simulink model "bit32cpu"  (R2020a)
settings: Solver=VariableStepAuto  StartTime=0.0  StopTime=10.0  RelTol=1e-3
libraries: simulink_extras x392
(part 7 of 63)

== system bit32cpu/ALU/Subsystem7/Subsystem2/Subsystem1 ==
  In1 : Inport
  In2 : Inport  Port=2
  In3 : Inport  Port=3
  In4 : Inport  Port=4
  In5 : Inport  Port=5
  In7 : Inport  Port=6
  In6 : Inport  Port=7
  Demux{,1..3} (4 alike) : Demux  Outputs=8
  Mux : Mux  Inputs=8
  Subsystem : Subsystem
  Subsystem1 : Subsystem
  Subsystem2 : Subsystem
  Subsystem3 : Subsystem
  Subsystem4 : Subsystem
  Subsystem5 : Subsystem
  Subsystem6 : Subsystem
  Subsystem7 : Subsystem
  Out1 : Outport
  wires:
  Demux3/7 -> Subsystem6/6(In6)
  In6/1 -> Subsystem4/7(In7), Subsystem7/7(In7), Subsystem5/7(In7), Subsystem6/7(In7), Subsystem1/7(In7), Subsystem3/7(In7), Subsystem2/7(In7), Subsystem/7(In7)
  Subsystem3/1(Out1) -> Mux/4
  Demux/1 -> Subsystem/3(In3)
  Demux2/8 -> Subsystem7/5(In5)
  Subsystem1/1(Out1) -> Mux/2
  Subsystem2/1(Out1) -> Mux/3
  Subsystem4/1(Out1) -> Mux/5
  Demux1/2 -> Subsystem1/4(In4)
  Demux/6 -> Subsystem5/3(In3)
  In4/1 -> Demux1/1
  Demux2/7 -> Subsystem6/5(In5)
  In3/1 -> Demux/1
  Demux1/4 -> Subsystem3/4(In4)
  In2/1 -> Subsystem4/2(In2), Subsystem5/2(In2), Subsystem6/2(In2), Subsystem7/2(In2), Subsystem2/2(In2), Subsystem3/2(In2), Subsystem/2(In2), Subsystem1/2(In2)
  Demux3/3 -> Subsystem2/6(In6)
  Subsystem/1(Out1) -> Mux/1
  Subsystem5/1(Out1) -> Mux/6
  In7/1 -> Demux3/1
  Mux/1 -> Out1/1
  Demux/3 -> Subsystem2/3(In3)
  Demux1/8 -> Subsystem7/4(In4)
  Demux3/6 -> Subsystem5/6(In6)
  Demux3/1 -> Subsystem/6(In6)
  Demux3/2 -> Subsystem1/6(In6)
  Subsystem6/1(Out1) -> Mux/7
  Demux1/3 -> Subsystem2/4(In4)
  Demux2/4 -> Subsystem3/5(In5)
  Demux1/5 -> Subsystem4/4(In4)
  In1/1 -> Subsystem6/1(In1), Subsystem7/1(In1), Subsystem4/1(In1), Subsystem5/1(In1), Subsystem2/1(In1), Subsystem3/1(In1), Subsystem/1(In1), Subsystem1/1(In1)
  Demux1/1 -> Subsystem/4(In4)
  Demux3/4 -> Subsystem3/6(In6)
  Demux2/2 -> Subsystem1/5(In5)
  Demux2/6 -> Subsystem5/5(In5)
  Demux/2 -> Subsystem1/3(In3)
  Demux/7 -> Subsystem6/3(In3)
  Demux3/8 -> Subsystem7/6(In6)
  Demux1/6 -> Subsystem5/4(In4)
  Demux/5 -> Subsystem4/3(In3)
  Demux2/5 -> Subsystem4/5(In5)
  Demux/8 -> Subsystem7/3(In3)
  Demux2/3 -> Subsystem2/5(In5)
  Demux3/5 -> Subsystem4/6(In6)
  In5/1 -> Demux2/1
  Demux1/7 -> Subsystem6/4(In4)
  Subsystem7/1(Out1) -> Mux/8
  Demux/4 -> Subsystem3/3(In3)
  Demux2/1 -> Subsystem/5(In5)

== system bit32cpu/ALU/Subsystem7/Subsystem2/Subsystem2 ==
  In1 : Inport
  In2 : Inport  Port=2
  In3 : Inport  Port=3
  In4 : Inport  Port=4
  In5 : Inport  Port=5
  In7 : Inport  Port=6
  In6 : Inport  Port=7
  Demux{,1..3} (4 alike) : Demux  Outputs=8
  Mux : Mux  Inputs=8
  Subsystem : Subsystem
  Subsystem1 : Subsystem
  Subsystem2 : Subsystem
  Subsystem3 : Subsystem
  Subsystem4 : Subsystem
  Subsystem5 : Subsystem
  Subsystem6 : Subsystem
  Subsystem7 : Subsystem
  Out1 : Outport
  wires:
  Demux3/7 -> Subsystem6/6(In6)
  In6/1 -> Subsystem4/7(In7), Subsystem7/7(In7), Subsystem5/7(In7), Subsystem6/7(In7), Subsystem1/7(In7), Subsystem3/7(In7), Subsystem2/7(In7), Subsystem/7(In7)
  Subsystem3/1(Out1) -> Mux/4
  Demux/1 -> Subsystem/3(In3)
  Demux2/8 -> Subsystem7/5(In5)
  Subsystem1/1(Out1) -> Mux/2
  Subsystem2/1(Out1) -> Mux/3
  Subsystem4/1(Out1) -> Mux/5
  Demux1/2 -> Subsystem1/4(In4)
  Demux/6 -> Subsystem5/3(In3)
  In4/1 -> Demux1/1
  Demux2/7 -> Subsystem6/5(In5)
  In3/1 -> Demux/1
  Demux1/4 -> Subsystem3/4(In4)
  In2/1 -> Subsystem4/2(In2), Subsystem5/2(In2), Subsystem6/2(In2), Subsystem7/2(In2), Subsystem2/2(In2), Subsystem3/2(In2), Subsystem/2(In2), Subsystem1/2(In2)
  Demux3/3 -> Subsystem2/6(In6)
  Subsystem/1(Out1) -> Mux/1
  Subsystem5/1(Out1) -> Mux/6
  In7/1 -> Demux3/1
  Mux/1 -> Out1/1
  Demux/3 -> Subsystem2/3(In3)
  Demux1/8 -> Subsystem7/4(In4)
  Demux3/6 -> Subsystem5/6(In6)
  Demux3/1 -> Subsystem/6(In6)
  Demux3/2 -> Subsystem1/6(In6)
  Subsystem6/1(Out1) -> Mux/7
  Demux1/3 -> Subsystem2/4(In4)
  Demux2/4 -> Subsystem3/5(In5)
  Demux1/5 -> Subsystem4/4(In4)
  In1/1 -> Subsystem6/1(In1), Subsystem7/1(In1), Subsystem4/1(In1), Subsystem5/1(In1), Subsystem2/1(In1), Subsystem3/1(In1), Subsystem/1(In1), Subsystem1/1(In1)
  Demux1/1 -> Subsystem/4(In4)
  Demux3/4 -> Subsystem3/6(In6)
  Demux2/2 -> Subsystem1/5(In5)
  Demux2/6 -> Subsystem5/5(In5)
  Demux/2 -> Subsystem1/3(In3)
  Demux/7 -> Subsystem6/3(In3)
  Demux3/8 -> Subsystem7/6(In6)
  Demux1/6 -> Subsystem5/4(In4)
  Demux/5 -> Subsystem4/3(In3)
  Demux2/5 -> Subsystem4/5(In5)
  Demux/8 -> Subsystem7/3(In3)
  Demux2/3 -> Subsystem2/5(In5)
  Demux3/5 -> Subsystem4/6(In6)
  In5/1 -> Demux2/1
  Demux1/7 -> Subsystem6/4(In4)
  Subsystem7/1(Out1) -> Mux/8
  Demux/4 -> Subsystem3/3(In3)
  Demux2/1 -> Subsystem/5(In5)

== system bit32cpu/ALU/Subsystem7/Subsystem2/Subsystem3 ==
  In1 : Inport
  In2 : Inport  Port=2
  In3 : Inport  Port=3
  In4 : Inport  Port=4
  In5 : Inport  Port=5
  In7 : Inport  Port=6
  In6 : Inport  Port=7
  Demux{,1..3} (4 alike) : Demux  Outputs=8
  Mux : Mux  Inputs=8
  Subsystem : Subsystem
  Subsystem1 : Subsystem
  Subsystem2 : Subsystem
  Subsystem3 : Subsystem
  Subsystem4 : Subsystem
  Subsystem5 : Subsystem
  Subsystem6 : Subsystem
  Subsystem7 : Subsystem
  Out1 : Outport
  wires:
  Demux3/7 -> Subsystem6/6(In6)
  In6/1 -> Subsystem4/7(In7), Subsystem7/7(In7), Subsystem5/7(In7), Subsystem6/7(In7), Subsystem1/7(In7), Subsystem3/7(In7), Subsystem2/7(In7), Subsystem/7(In7)
  Subsystem3/1(Out1) -> Mux/4
  Demux/1 -> Subsystem/3(In3)
  Demux2/8 -> Subsystem7/5(In5)
  Subsystem1/1(Out1) -> Mux/2
  Subsystem2/1(Out1) -> Mux/3
  Subsystem4/1(Out1) -> Mux/5
  Demux1/2 -> Subsystem1/4(In4)
  Demux/6 -> Subsystem5/3(In3)
  In4/1 -> Demux1/1
  Demux2/7 -> Subsystem6/5(In5)
  In3/1 -> Demux/1
  Demux1/4 -> Subsystem3/4(In4)
  In2/1 -> Subsystem4/2(In2), Subsystem5/2(In2), Subsystem6/2(In2), Subsystem7/2(In2), Subsystem2/2(In2), Subsystem3/2(In2), Subsystem/2(In2), Subsystem1/2(In2)
  Demux3/3 -> Subsystem2/6(In6)
  Subsystem/1(Out1) -> Mux/1
  Subsystem5/1(Out1) -> Mux/6
  In7/1 -> Demux3/1
  Mux/1 -> Out1/1
  Demux/3 -> Subsystem2/3(In3)
  Demux1/8 -> Subsystem7/4(In4)
  Demux3/6 -> Subsystem5/6(In6)
  Demux3/1 -> Subsystem/6(In6)
  Demux3/2 -> Subsystem1/6(In6)
  Subsystem6/1(Out1) -> Mux/7
  Demux1/3 -> Subsystem2/4(In4)
  Demux2/4 -> Subsystem3/5(In5)
  Demux1/5 -> Subsystem4/4(In4)
  In1/1 -> Subsystem6/1(In1), Subsystem7/1(In1), Subsystem4/1(In1), Subsystem5/1(In1), Subsystem2/1(In1), Subsystem3/1(In1), Subsystem/1(In1), Subsystem1/1(In1)
  Demux1/1 -> Subsystem/4(In4)
  Demux3/4 -> Subsystem3/6(In6)
  Demux2/2 -> Subsystem1/5(In5)
  Demux2/6 -> Subsystem5/5(In5)
  Demux/2 -> Subsystem1/3(In3)
  Demux/7 -> Subsystem6/3(In3)
  Demux3/8 -> Subsystem7/6(In6)
  Demux1/6 -> Subsystem5/4(In4)
  Demux/5 -> Subsystem4/3(In3)
  Demux2/5 -> Subsystem4/5(In5)
  Demux/8 -> Subsystem7/3(In3)
  Demux2/3 -> Subsystem2/5(In5)
  Demux3/5 -> Subsystem4/6(In6)
  In5/1 -> Demux2/1
  Demux1/7 -> Subsystem6/4(In4)
  Subsystem7/1(Out1) -> Mux/8
  Demux/4 -> Subsystem3/3(In3)
  Demux2/1 -> Subsystem/5(In5)

== system bit32cpu/ALU/Subsystem7/Subsystem2/Subsystem4 ==
  In1 : Inport
  In2 : Inport  Port=2
  In3 : Inport  Port=3
  In4 : Inport  Port=4
  In5 : Inport  Port=5
  In7 : Inport  Port=6
  In6 : Inport  Port=7
  Demux{,1..3} (4 alike) : Demux  Outputs=8
  Mux : Mux  Inputs=8
  Subsystem : Subsystem
  Subsystem1 : Subsystem
  Subsystem2 : Subsystem
  Subsystem3 : Subsystem
  Subsystem4 : Subsystem
  Subsystem5 : Subsystem
  Subsystem6 : Subsystem
  Subsystem7 : Subsystem
  Out1 : Outport
  wires:
  Demux3/7 -> Subsystem6/6(In6)
  In6/1 -> Subsystem4/7(In7), Subsystem7/7(In7), Subsystem5/7(In7), Subsystem6/7(In7), Subsystem1/7(In7), Subsystem3/7(In7), Subsystem2/7(In7), Subsystem/7(In7)
  Subsystem3/1(Out1) -> Mux/4
  Demux/1 -> Subsystem/3(In3)
  Demux2/8 -> Subsystem7/5(In5)
  Subsystem1/1(Out1) -> Mux/2
  Subsystem2/1(Out1) -> Mux/3
  Subsystem4/1(Out1) -> Mux/5
  Demux1/2 -> Subsystem1/4(In4)
  Demux/6 -> Subsystem5/3(In3)
  In4/1 -> Demux1/1
  Demux2/7 -> Subsystem6/5(In5)
  In3/1 -> Demux/1
  Demux1/4 -> Subsystem3/4(In4)
  In2/1 -> Subsystem4/2(In2), Subsystem5/2(In2), Subsystem6/2(In2), Subsystem7/2(In2), Subsystem2/2(In2), Subsystem3/2(In2), Subsystem/2(In2), Subsystem1/2(In2)
  Demux3/3 -> Subsystem2/6(In6)
  Subsystem/1(Out1) -> Mux/1
  Subsystem5/1(Out1) -> Mux/6
  In7/1 -> Demux3/1
  Mux/1 -> Out1/1
  Demux/3 -> Subsystem2/3(In3)
  Demux1/8 -> Subsystem7/4(In4)
  Demux3/6 -> Subsystem5/6(In6)
  Demux3/1 -> Subsystem/6(In6)
  Demux3/2 -> Subsystem1/6(In6)
  Subsystem6/1(Out1) -> Mux/7
  Demux1/3 -> Subsystem2/4(In4)
  Demux2/4 -> Subsystem3/5(In5)
  Demux1/5 -> Subsystem4/4(In4)
  In1/1 -> Subsystem6/1(In1), Subsystem7/1(In1), Subsystem4/1(In1), Subsystem5/1(In1), Subsystem2/1(In1), Subsystem3/1(In1), Subsystem/1(In1), Subsystem1/1(In1)
  Demux1/1 -> Subsystem/4(In4)
  Demux3/4 -> Subsystem3/6(In6)
  Demux2/2 -> Subsystem1/5(In5)
  Demux2/6 -> Subsystem5/5(In5)
  Demux/2 -> Subsystem1/3(In3)
  Demux/7 -> Subsystem6/3(In3)
  Demux3/8 -> Subsystem7/6(In6)
  Demux1/6 -> Subsystem5/4(In4)
  Demux/5 -> Subsystem4/3(In3)
  Demux2/5 -> Subsystem4/5(In5)
  Demux/8 -> Subsystem7/3(In3)
  Demux2/3 -> Subsystem2/5(In5)
  Demux3/5 -> Subsystem4/6(In6)
  In5/1 -> Demux2/1
  Demux1/7 -> Subsystem6/4(In4)
  Subsystem7/1(Out1) -> Mux/8
  Demux/4 -> Subsystem3/3(In3)
  Demux2/1 -> Subsystem/5(In5)

== system bit32cpu/ALU/Subsystem7/Subsystem2/Subsystem5 ==
  In1 : Inport
  In2 : Inport  Port=2
  In3 : Inport  Port=3
  In4 : Inport  Port=4
  In5 : Inport  Port=5
  In7 : Inport  Port=6
  In6 : Inport  Port=7
  Demux{,1..3} (4 alike) : Demux  Outputs=8
  Mux : Mux  Inputs=8
  Subsystem : Subsystem
  Subsystem1 : Subsystem
  Subsystem2 : Subsystem
  Subsystem3 : Subsystem
  Subsystem4 : Subsystem
  Subsystem5 : Subsystem
  Subsystem6 : Subsystem
  Subsystem7 : Subsystem
  Out1 : Outport
  wires:
  Demux3/7 -> Subsystem6/6(In6)
  In6/1 -> Subsystem4/7(In7), Subsystem7/7(In7), Subsystem5/7(In7), Subsystem6/7(In7), Subsystem1/7(In7), Subsystem3/7(In7), Subsystem2/7(In7), Subsystem/7(In7)
  Subsystem3/1(Out1) -> Mux/4
  Demux/1 -> Subsystem/3(In3)
  Demux2/8 -> Subsystem7/5(In5)
  Subsystem1/1(Out1) -> Mux/2
  Subsystem2/1(Out1) -> Mux/3
  Subsystem4/1(Out1) -> Mux/5
  Demux1/2 -> Subsystem1/4(In4)
  Demux/6 -> Subsystem5/3(In3)
  In4/1 -> Demux1/1
  Demux2/7 -> Subsystem6/5(In5)
  In3/1 -> Demux/1
  Demux1/4 -> Subsystem3/4(In4)
  In2/1 -> Subsystem4/2(In2), Subsystem5/2(In2), Subsystem6/2(In2), Subsystem7/2(In2), Subsystem2/2(In2), Subsystem3/2(In2), Subsystem/2(In2), Subsystem1/2(In2)
  Demux3/3 -> Subsystem2/6(In6)
  Subsystem/1(Out1) -> Mux/1
  Subsystem5/1(Out1) -> Mux/6
  In7/1 -> Demux3/1
  Mux/1 -> Out1/1
  Demux/3 -> Subsystem2/3(In3)
  Demux1/8 -> Subsystem7/4(In4)
  Demux3/6 -> Subsystem5/6(In6)
  Demux3/1 -> Subsystem/6(In6)
  Demux3/2 -> Subsystem1/6(In6)
  Subsystem6/1(Out1) -> Mux/7
  Demux1/3 -> Subsystem2/4(In4)
  Demux2/4 -> Subsystem3/5(In5)
  Demux1/5 -> Subsystem4/4(In4)
  In1/1 -> Subsystem6/1(In1), Subsystem7/1(In1), Subsystem4/1(In1), Subsystem5/1(In1), Subsystem2/1(In1), Subsystem3/1(In1), Subsystem/1(In1), Subsystem1/1(In1)
  Demux1/1 -> Subsystem/4(In4)
  Demux3/4 -> Subsystem3/6(In6)
  Demux2/2 -> Subsystem1/5(In5)
  Demux2/6 -> Subsystem5/5(In5)
  Demux/2 -> Subsystem1/3(In3)
  Demux/7 -> Subsystem6/3(In3)
  Demux3/8 -> Subsystem7/6(In6)
  Demux1/6 -> Subsystem5/4(In4)
  Demux/5 -> Subsystem4/3(In3)
  Demux2/5 -> Subsystem4/5(In5)
  Demux/8 -> Subsystem7/3(In3)
  Demux2/3 -> Subsystem2/5(In5)
  Demux3/5 -> Subsystem4/6(In6)
  In5/1 -> Demux2/1
  Demux1/7 -> Subsystem6/4(In4)
  Subsystem7/1(Out1) -> Mux/8
  Demux/4 -> Subsystem3/3(In3)
  Demux2/1 -> Subsystem/5(In5)

== system bit32cpu/ALU/Subsystem7/Subsystem3/Subsystem1 ==
  In1 : Inport
  In2 : Inport  Port=2
  In3 : Inport  Port=3
  In4 : Inport  Port=4
  In5 : Inport  Port=5
  In7 : Inport  Port=6
  In6 : Inport  Port=7
  Demux{,1..3} (4 alike) : Demux  Outputs=8
  Mux : Mux  Inputs=8
  Subsystem : Subsystem
  Subsystem1 : Subsystem
  Subsystem2 : Subsystem
  Subsystem3 : Subsystem
  Subsystem4 : Subsystem
  Subsystem5 : Subsystem
  Subsystem6 : Subsystem
  Subsystem7 : Subsystem
  Out1 : Outport
  wires:
  Demux3/7 -> Subsystem6/6(In6)
  In6/1 -> Subsystem4/7(In7), Subsystem7/7(In7), Subsystem5/7(In7), Subsystem6/7(In7), Subsystem1/7(In7), Subsystem3/7(In7), Subsystem2/7(In7), Subsystem/7(In7)
  Subsystem3/1(Out1) -> Mux/4
  Demux/1 -> Subsystem/3(In3)
  Demux2/8 -> Subsystem7/5(In5)
  Subsystem1/1(Out1) -> Mux/2
  Subsystem2/1(Out1) -> Mux/3
  Subsystem4/1(Out1) -> Mux/5
  Demux1/2 -> Subsystem1/4(In4)
  Demux/6 -> Subsystem5/3(In3)
  In4/1 -> Demux1/1
  Demux2/7 -> Subsystem6/5(In5)
  In3/1 -> Demux/1
  Demux1/4 -> Subsystem3/4(In4)
  In2/1 -> Subsystem4/2(In2), Subsystem5/2(In2), Subsystem6/2(In2), Subsystem7/2(In2), Subsystem2/2(In2), Subsystem3/2(In2), Subsystem/2(In2), Subsystem1/2(In2)
  Demux3/3 -> Subsystem2/6(In6)
  Subsystem/1(Out1) -> Mux/1
  Subsystem5/1(Out1) -> Mux/6
  In7/1 -> Demux3/1
  Mux/1 -> Out1/1
  Demux/3 -> Subsystem2/3(In3)
  Demux1/8 -> Subsystem7/4(In4)
  Demux3/6 -> Subsystem5/6(In6)
  Demux3/1 -> Subsystem/6(In6)
  Demux3/2 -> Subsystem1/6(In6)
  Subsystem6/1(Out1) -> Mux/7
  Demux1/3 -> Subsystem2/4(In4)
  Demux2/4 -> Subsystem3/5(In5)
  Demux1/5 -> Subsystem4/4(In4)
  In1/1 -> Subsystem6/1(In1), Subsystem7/1(In1), Subsystem4/1(In1), Subsystem5/1(In1), Subsystem2/1(In1), Subsystem3/1(In1), Subsystem/1(In1), Subsystem1/1(In1)
  Demux1/1 -> Subsystem/4(In4)
  Demux3/4 -> Subsystem3/6(In6)
  Demux2/2 -> Subsystem1/5(In5)
  Demux2/6 -> Subsystem5/5(In5)
  Demux/2 -> Subsystem1/3(In3)
  Demux/7 -> Subsystem6/3(In3)
  Demux3/8 -> Subsystem7/6(In6)
  Demux1/6 -> Subsystem5/4(In4)
  Demux/5 -> Subsystem4/3(In3)
  Demux2/5 -> Subsystem4/5(In5)
  Demux/8 -> Subsystem7/3(In3)
  Demux2/3 -> Subsystem2/5(In5)
  Demux3/5 -> Subsystem4/6(In6)
  In5/1 -> Demux2/1
  Demux1/7 -> Subsystem6/4(In4)
  Subsystem7/1(Out1) -> Mux/8
  Demux/4 -> Subsystem3/3(In3)
  Demux2/1 -> Subsystem/5(In5)

== system bit32cpu/ALU/Subsystem7/Subsystem3/Subsystem2 ==
  In1 : Inport
  In2 : Inport  Port=2
  In3 : Inport  Port=3
  In4 : Inport  Port=4
  In5 : Inport  Port=5
  In7 : Inport  Port=6
  In6 : Inport  Port=7
  Demux{,1..3} (4 alike) : Demux  Outputs=8
  Mux : Mux  Inputs=8
  Subsystem : Subsystem
  Subsystem1 : Subsystem
  Subsystem2 : Subsystem
  Subsystem3 : Subsystem
  Subsystem4 : Subsystem
  Subsystem5 : Subsystem
  Subsystem6 : Subsystem
  Subsystem7 : Subsystem
  Out1 : Outport
  wires:
  Demux3/7 -> Subsystem6/6(In6)
  In6/1 -> Subsystem4/7(In7), Subsystem7/7(In7), Subsystem5/7(In7), Subsystem6/7(In7), Subsystem1/7(In7), Subsystem3/7(In7), Subsystem2/7(In7), Subsystem/7(In7)
  Subsystem3/1(Out1) -> Mux/4
  Demux/1 -> Subsystem/3(In3)
  Demux2/8 -> Subsystem7/5(In5)
  Subsystem1/1(Out1) -> Mux/2
  Subsystem2/1(Out1) -> Mux/3
  Subsystem4/1(Out1) -> Mux/5
  Demux1/2 -> Subsystem1/4(In4)
  Demux/6 -> Subsystem5/3(In3)
  In4/1 -> Demux1/1
  Demux2/7 -> Subsystem6/5(In5)
  In3/1 -> Demux/1
  Demux1/4 -> Subsystem3/4(In4)
  In2/1 -> Subsystem4/2(In2), Subsystem5/2(In2), Subsystem6/2(In2), Subsystem7/2(In2), Subsystem2/2(In2), Subsystem3/2(In2), Subsystem/2(In2), Subsystem1/2(In2)
  Demux3/3 -> Subsystem2/6(In6)
  Subsystem/1(Out1) -> Mux/1
  Subsystem5/1(Out1) -> Mux/6
  In7/1 -> Demux3/1
  Mux/1 -> Out1/1
  Demux/3 -> Subsystem2/3(In3)
  Demux1/8 -> Subsystem7/4(In4)
  Demux3/6 -> Subsystem5/6(In6)
  Demux3/1 -> Subsystem/6(In6)
  Demux3/2 -> Subsystem1/6(In6)
  Subsystem6/1(Out1) -> Mux/7
  Demux1/3 -> Subsystem2/4(In4)
  Demux2/4 -> Subsystem3/5(In5)
  Demux1/5 -> Subsystem4/4(In4)
  In1/1 -> Subsystem6/1(In1), Subsystem7/1(In1), Subsystem4/1(In1), Subsystem5/1(In1), Subsystem2/1(In1), Subsystem3/1(In1), Subsystem/1(In1), Subsystem1/1(In1)
  Demux1/1 -> Subsystem/4(In4)
  Demux3/4 -> Subsystem3/6(In6)
  Demux2/2 -> Subsystem1/5(In5)
  Demux2/6 -> Subsystem5/5(In5)
  Demux/2 -> Subsystem1/3(In3)
  Demux/7 -> Subsystem6/3(In3)
  Demux3/8 -> Subsystem7/6(In6)
  Demux1/6 -> Subsystem5/4(In4)
  Demux/5 -> Subsystem4/3(In3)
  Demux2/5 -> Subsystem4/5(In5)
  Demux/8 -> Subsystem7/3(In3)
  Demux2/3 -> Subsystem2/5(In5)
  Demux3/5 -> Subsystem4/6(In6)
  In5/1 -> Demux2/1
  Demux1/7 -> Subsystem6/4(In4)
  Subsystem7/1(Out1) -> Mux/8
  Demux/4 -> Subsystem3/3(In3)
  Demux2/1 -> Subsystem/5(In5)

== system bit32cpu/ALU/Subsystem7/Subsystem3/Subsystem3 ==
  In1 : Inport
  In2 : Inport  Port=2
  In3 : Inport  Port=3
  In4 : Inport  Port=4
  In5 : Inport  Port=5
  In7 : Inport  Port=6
  In6 : Inport  Port=7
  Demux{,1..3} (4 alike) : Demux  Outputs=8
  Mux : Mux  Inputs=8
  Subsystem : Subsystem
  Subsystem1 : Subsystem
  Subsystem2 : Subsystem
  Subsystem3 : Subsystem
  Subsystem4 : Subsystem
  Subsystem5 : Subsystem
  Subsystem6 : Subsystem
  Subsystem7 : Subsystem
  Out1 : Outport
  wires:
  Demux3/7 -> Subsystem6/6(In6)
  In6/1 -> Subsystem4/7(In7), Subsystem7/7(In7), Subsystem5/7(In7), Subsystem6/7(In7), Subsystem1/7(In7), Subsystem3/7(In7), Subsystem2/7(In7), Subsystem/7(In7)
  Subsystem3/1(Out1) -> Mux/4
  Demux/1 -> Subsystem/3(In3)
  Demux2/8 -> Subsystem7/5(In5)
  Subsystem1/1(Out1) -> Mux/2
  Subsystem2/1(Out1) -> Mux/3
  Subsystem4/1(Out1) -> Mux/5
  Demux1/2 -> Subsystem1/4(In4)
  Demux/6 -> Subsystem5/3(In3)
  In4/1 -> Demux1/1
  Demux2/7 -> Subsystem6/5(In5)
  In3/1 -> Demux/1
  Demux1/4 -> Subsystem3/4(In4)
  In2/1 -> Subsystem4/2(In2), Subsystem5/2(In2), Subsystem6/2(In2), Subsystem7/2(In2), Subsystem2/2(In2), Subsystem3/2(In2), Subsystem/2(In2), Subsystem1/2(In2)
  Demux3/3 -> Subsystem2/6(In6)
  Subsystem/1(Out1) -> Mux/1
  Subsystem5/1(Out1) -> Mux/6
  In7/1 -> Demux3/1
  Mux/1 -> Out1/1
  Demux/3 -> Subsystem2/3(In3)
  Demux1/8 -> Subsystem7/4(In4)
  Demux3/6 -> Subsystem5/6(In6)
  Demux3/1 -> Subsystem/6(In6)
  Demux3/2 -> Subsystem1/6(In6)
  Subsystem6/1(Out1) -> Mux/7
  Demux1/3 -> Subsystem2/4(In4)
  Demux2/4 -> Subsystem3/5(In5)
  Demux1/5 -> Subsystem4/4(In4)
  In1/1 -> Subsystem6/1(In1), Subsystem7/1(In1), Subsystem4/1(In1), Subsystem5/1(In1), Subsystem2/1(In1), Subsystem3/1(In1), Subsystem/1(In1), Subsystem1/1(In1)
  Demux1/1 -> Subsystem/4(In4)
  Demux3/4 -> Subsystem3/6(In6)
  Demux2/2 -> Subsystem1/5(In5)
  Demux2/6 -> Subsystem5/5(In5)
  Demux/2 -> Subsystem1/3(In3)
  Demux/7 -> Subsystem6/3(In3)
  Demux3/8 -> Subsystem7/6(In6)
  Demux1/6 -> Subsystem5/4(In4)
  Demux/5 -> Subsystem4/3(In3)
  Demux2/5 -> Subsystem4/5(In5)
  Demux/8 -> Subsystem7/3(In3)
  Demux2/3 -> Subsystem2/5(In5)
  Demux3/5 -> Subsystem4/6(In6)
  In5/1 -> Demux2/1
  Demux1/7 -> Subsystem6/4(In4)
  Subsystem7/1(Out1) -> Mux/8
  Demux/4 -> Subsystem3/3(In3)
  Demux2/1 -> Subsystem/5(In5)

== system bit32cpu/ALU/Subsystem7/Subsystem3/Subsystem4 ==
  In1 : Inport
  In2 : Inport  Port=2
  In3 : Inport  Port=3
  In4 : Inport  Port=4
  In5 : Inport  Port=5
  In7 : Inport  Port=6
  In6 : Inport  Port=7
  Demux{,1..3} (4 alike) : Demux  Outputs=8
  Mux : Mux  Inputs=8
  Subsystem : Subsystem
  Subsystem1 : Subsystem
  Subsystem2 : Subsystem
  Subsystem3 : Subsystem
  Subsystem4 : Subsystem
  Subsystem5 : Subsystem
  Subsystem6 : Subsystem
  Subsystem7 : Subsystem
  Out1 : Outport
  wires:
  Demux3/7 -> Subsystem6/6(In6)
  In6/1 -> Subsystem4/7(In7), Subsystem7/7(In7), Subsystem5/7(In7), Subsystem6/7(In7), Subsystem1/7(In7), Subsystem3/7(In7), Subsystem2/7(In7), Subsystem/7(In7)
  Subsystem3/1(Out1) -> Mux/4
  Demux/1 -> Subsystem/3(In3)
  Demux2/8 -> Subsystem7/5(In5)
  Subsystem1/1(Out1) -> Mux/2
  Subsystem2/1(Out1) -> Mux/3
  Subsystem4/1(Out1) -> Mux/5
  Demux1/2 -> Subsystem1/4(In4)
  Demux/6 -> Subsystem5/3(In3)
  In4/1 -> Demux1/1
  Demux2/7 -> Subsystem6/5(In5)
  In3/1 -> Demux/1
  Demux1/4 -> Subsystem3/4(In4)
  In2/1 -> Subsystem4/2(In2), Subsystem5/2(In2), Subsystem6/2(In2), Subsystem7/2(In2), Subsystem2/2(In2), Subsystem3/2(In2), Subsystem/2(In2), Subsystem1/2(In2)
  Demux3/3 -> Subsystem2/6(In6)
  Subsystem/1(Out1) -> Mux/1
  Subsystem5/1(Out1) -> Mux/6
  In7/1 -> Demux3/1
  Mux/1 -> Out1/1
  Demux/3 -> Subsystem2/3(In3)
  Demux1/8 -> Subsystem7/4(In4)
  Demux3/6 -> Subsystem5/6(In6)
  Demux3/1 -> Subsystem/6(In6)
  Demux3/2 -> Subsystem1/6(In6)
  Subsystem6/1(Out1) -> Mux/7
  Demux1/3 -> Subsystem2/4(In4)
  Demux2/4 -> Subsystem3/5(In5)
  Demux1/5 -> Subsystem4/4(In4)
  In1/1 -> Subsystem6/1(In1), Subsystem7/1(In1), Subsystem4/1(In1), Subsystem5/1(In1), Subsystem2/1(In1), Subsystem3/1(In1), Subsystem/1(In1), Subsystem1/1(In1)
  Demux1/1 -> Subsystem/4(In4)
  Demux3/4 -> Subsystem3/6(In6)
  Demux2/2 -> Subsystem1/5(In5)
  Demux2/6 -> Subsystem5/5(In5)
  Demux/2 -> Subsystem1/3(In3)
  Demux/7 -> Subsystem6/3(In3)
  Demux3/8 -> Subsystem7/6(In6)
  Demux1/6 -> Subsystem5/4(In4)
  Demux/5 -> Subsystem4/3(In3)
  Demux2/5 -> Subsystem4/5(In5)
  Demux/8 -> Subsystem7/3(In3)
  Demux2/3 -> Subsystem2/5(In5)
  Demux3/5 -> Subsystem4/6(In6)
  In5/1 -> Demux2/1
  Demux1/7 -> Subsystem6/4(In4)
  Subsystem7/1(Out1) -> Mux/8
  Demux/4 -> Subsystem3/3(In3)
  Demux2/1 -> Subsystem/5(In5)

== system bit32cpu/ALU/Subsystem7/Subsystem3/Subsystem5 ==
  In1 : Inport
  In2 : Inport  Port=2
  In3 : Inport  Port=3
  In4 : Inport  Port=4
  In5 : Inport  Port=5
  In7 : Inport  Port=6
  In6 : Inport  Port=7
  Demux{,1..3} (4 alike) : Demux  Outputs=8
  Mux : Mux  Inputs=8
  Subsystem : Subsystem
  Subsystem1 : Subsystem
  Subsystem2 : Subsystem
  Subsystem3 : Subsystem
  Subsystem4 : Subsystem
  Subsystem5 : Subsystem
  Subsystem6 : Subsystem
  Subsystem7 : Subsystem
  Out1 : Outport
  wires:
  Demux3/7 -> Subsystem6/6(In6)
  In6/1 -> Subsystem4/7(In7), Subsystem7/7(In7), Subsystem5/7(In7), Subsystem6/7(In7), Subsystem1/7(In7), Subsystem3/7(In7), Subsystem2/7(In7), Subsystem/7(In7)
  Subsystem3/1(Out1) -> Mux/4
  Demux/1 -> Subsystem/3(In3)
  Demux2/8 -> Subsystem7/5(In5)
  Subsystem1/1(Out1) -> Mux/2
  Subsystem2/1(Out1) -> Mux/3
  Subsystem4/1(Out1) -> Mux/5
  Demux1/2 -> Subsystem1/4(In4)
  Demux/6 -> Subsystem5/3(In3)
  In4/1 -> Demux1/1
  Demux2/7 -> Subsystem6/5(In5)
  In3/1 -> Demux/1
  Demux1/4 -> Subsystem3/4(In4)
  In2/1 -> Subsystem4/2(In2), Subsystem5/2(In2), Subsystem6/2(In2), Subsystem7/2(In2), Subsystem2/2(In2), Subsystem3/2(In2), Subsystem/2(In2), Subsystem1/2(In2)
  Demux3/3 -> Subsystem2/6(In6)
  Subsystem/1(Out1) -> Mux/1
  Subsystem5/1(Out1) -> Mux/6
  In7/1 -> Demux3/1
  Mux/1 -> Out1/1
  Demux/3 -> Subsystem2/3(In3)
  Demux1/8 -> Subsystem7/4(In4)
  Demux3/6 -> Subsystem5/6(In6)
  Demux3/1 -> Subsystem/6(In6)
  Demux3/2 -> Subsystem1/6(In6)
  Subsystem6/1(Out1) -> Mux/7
  Demux1/3 -> Subsystem2/4(In4)
  Demux2/4 -> Subsystem3/5(In5)
  Demux1/5 -> Subsystem4/4(In4)
  In1/1 -> Subsystem6/1(In1), Subsystem7/1(In1), Subsystem4/1(In1), Subsystem5/1(In1), Subsystem2/1(In1), Subsystem3/1(In1), Subsystem/1(In1), Subsystem1/1(In1)
  Demux1/1 -> Subsystem/4(In4)
  Demux3/4 -> Subsystem3/6(In6)
  Demux2/2 -> Subsystem1/5(In5)
  Demux2/6 -> Subsystem5/5(In5)
  Demux/2 -> Subsystem1/3(In3)
  Demux/7 -> Subsystem6/3(In3)
  Demux3/8 -> Subsystem7/6(In6)
  Demux1/6 -> Subsystem5/4(In4)
  Demux/5 -> Subsystem4/3(In3)
  Demux2/5 -> Subsystem4/5(In5)
  Demux/8 -> Subsystem7/3(In3)
  Demux2/3 -> Subsystem2/5(In5)
  Demux3/5 -> Subsystem4/6(In6)
  In5/1 -> Demux2/1
  Demux1/7 -> Subsystem6/4(In4)
  Subsystem7/1(Out1) -> Mux/8
  Demux/4 -> Subsystem3/3(In3)
  Demux2/1 -> Subsystem/5(In5)

== system bit32cpu/ALU/Subsystem7/Subsystem4/Subsystem1 ==
  In1 : Inport
  In2 : Inport  Port=2
  In3 : Inport  Port=3
  In4 : Inport  Port=4
  In5 : Inport  Port=5
  In7 : Inport  Port=6
  In6 : Inport  Port=7
  Demux{,1..3} (4 alike) : Demux  Outputs=8
  Mux : Mux  Inputs=8
  Subsystem : Subsystem
  Subsystem1 : Subsystem
  Subsystem2 : Subsystem
  Subsystem3 : Subsystem
  Subsystem4 : Subsystem
  Subsystem5 : Subsystem
  Subsystem6 : Subsystem
  Subsystem7 : Subsystem
  Out1 : Outport
  wires:
  Demux3/7 -> Subsystem6/6(In6)
  In6/1 -> Subsystem4/7(In7), Subsystem7/7(In7), Subsystem5/7(In7), Subsystem6/7(In7), Subsystem1/7(In7), Subsystem3/7(In7), Subsystem2/7(In7), Subsystem/7(In7)
  Subsystem3/1(Out1) -> Mux/4
  Demux/1 -> Subsystem/3(In3)
  Demux2/8 -> Subsystem7/5(In5)
  Subsystem1/1(Out1) -> Mux/2
  Subsystem2/1(Out1) -> Mux/3
  Subsystem4/1(Out1) -> Mux/5
  Demux1/2 -> Subsystem1/4(In4)
  Demux/6 -> Subsystem5/3(In3)
  In4/1 -> Demux1/1
  Demux2/7 -> Subsystem6/5(In5)
  In3/1 -> Demux/1
  Demux1/4 -> Subsystem3/4(In4)
  In2/1 -> Subsystem4/2(In2), Subsystem5/2(In2), Subsystem6/2(In2), Subsystem7/2(In2), Subsystem2/2(In2), Subsystem3/2(In2), Subsystem/2(In2), Subsystem1/2(In2)
  Demux3/3 -> Subsystem2/6(In6)
  Subsystem/1(Out1) -> Mux/1
  Subsystem5/1(Out1) -> Mux/6
  In7/1 -> Demux3/1
  Mux/1 -> Out1/1
  Demux/3 -> Subsystem2/3(In3)
  Demux1/8 -> Subsystem7/4(In4)
  Demux3/6 -> Subsystem5/6(In6)
  Demux3/1 -> Subsystem/6(In6)
  Demux3/2 -> Subsystem1/6(In6)
  Subsystem6/1(Out1) -> Mux/7
  Demux1/3 -> Subsystem2/4(In4)
  Demux2/4 -> Subsystem3/5(In5)
  Demux1/5 -> Subsystem4/4(In4)
  In1/1 -> Subsystem6/1(In1), Subsystem7/1(In1), Subsystem4/1(In1), Subsystem5/1(In1), Subsystem2/1(In1), Subsystem3/1(In1), Subsystem/1(In1), Subsystem1/1(In1)
  Demux1/1 -> Subsystem/4(In4)
  Demux3/4 -> Subsystem3/6(In6)
  Demux2/2 -> Subsystem1/5(In5)
  Demux2/6 -> Subsystem5/5(In5)
  Demux/2 -> Subsystem1/3(In3)
  Demux/7 -> Subsystem6/3(In3)
  Demux3/8 -> Subsystem7/6(In6)
  Demux1/6 -> Subsystem5/4(In4)
  Demux/5 -> Subsystem4/3(In3)
  Demux2/5 -> Subsystem4/5(In5)
  Demux/8 -> Subsystem7/3(In3)
  Demux2/3 -> Subsystem2/5(In5)
  Demux3/5 -> Subsystem4/6(In6)
  In5/1 -> Demux2/1
  Demux1/7 -> Subsystem6/4(In4)
  Subsystem7/1(Out1) -> Mux/8
  Demux/4 -> Subsystem3/3(In3)
  Demux2/1 -> Subsystem/5(In5)

== system bit32cpu/ALU/Subsystem7/Subsystem4/Subsystem2 ==
  In1 : Inport
  In2 : Inport  Port=2
  In3 : Inport  Port=3
  In4 : Inport  Port=4
  In5 : Inport  Port=5
  In7 : Inport  Port=6
  In6 : Inport  Port=7
  Demux{,1..3} (4 alike) : Demux  Outputs=8
  Mux : Mux  Inputs=8
  Subsystem : Subsystem
  Subsystem1 : Subsystem
  Subsystem2 : Subsystem
  Subsystem3 : Subsystem
  Subsystem4 : Subsystem
  Subsystem5 : Subsystem
  Subsystem6 : Subsystem
  Subsystem7 : Subsystem
  Out1 : Outport
  wires:
  Demux3/7 -> Subsystem6/6(In6)
  In6/1 -> Subsystem4/7(In7), Subsystem7/7(In7), Subsystem5/7(In7), Subsystem6/7(In7), Subsystem1/7(In7), Subsystem3/7(In7), Subsystem2/7(In7), Subsystem/7(In7)
  Subsystem3/1(Out1) -> Mux/4
  Demux/1 -> Subsystem/3(In3)
  Demux2/8 -> Subsystem7/5(In5)
  Subsystem1/1(Out1) -> Mux/2
  Subsystem2/1(Out1) -> Mux/3
  Subsystem4/1(Out1) -> Mux/5
  Demux1/2 -> Subsystem1/4(In4)
  Demux/6 -> Subsystem5/3(In3)
  In4/1 -> Demux1/1
  Demux2/7 -> Subsystem6/5(In5)
  In3/1 -> Demux/1
  Demux1/4 -> Subsystem3/4(In4)
  In2/1 -> Subsystem4/2(In2), Subsystem5/2(In2), Subsystem6/2(In2), Subsystem7/2(In2), Subsystem2/2(In2), Subsystem3/2(In2), Subsystem/2(In2), Subsystem1/2(In2)
  Demux3/3 -> Subsystem2/6(In6)
  Subsystem/1(Out1) -> Mux/1
  Subsystem5/1(Out1) -> Mux/6
  In7/1 -> Demux3/1
  Mux/1 -> Out1/1
  Demux/3 -> Subsystem2/3(In3)
  Demux1/8 -> Subsystem7/4(In4)
  Demux3/6 -> Subsystem5/6(In6)
  Demux3/1 -> Subsystem/6(In6)
  Demux3/2 -> Subsystem1/6(In6)
  Subsystem6/1(Out1) -> Mux/7
  Demux1/3 -> Subsystem2/4(In4)
  Demux2/4 -> Subsystem3/5(In5)
  Demux1/5 -> Subsystem4/4(In4)
  In1/1 -> Subsystem6/1(In1), Subsystem7/1(In1), Subsystem4/1(In1), Subsystem5/1(In1), Subsystem2/1(In1), Subsystem3/1(In1), Subsystem/1(In1), Subsystem1/1(In1)
  Demux1/1 -> Subsystem/4(In4)
  Demux3/4 -> Subsystem3/6(In6)
  Demux2/2 -> Subsystem1/5(In5)
  Demux2/6 -> Subsystem5/5(In5)
  Demux/2 -> Subsystem1/3(In3)
  Demux/7 -> Subsystem6/3(In3)
  Demux3/8 -> Subsystem7/6(In6)
  Demux1/6 -> Subsystem5/4(In4)
  Demux/5 -> Subsystem4/3(In3)
  Demux2/5 -> Subsystem4/5(In5)
  Demux/8 -> Subsystem7/3(In3)
  Demux2/3 -> Subsystem2/5(In5)
  Demux3/5 -> Subsystem4/6(In6)
  In5/1 -> Demux2/1
  Demux1/7 -> Subsystem6/4(In4)
  Subsystem7/1(Out1) -> Mux/8
  Demux/4 -> Subsystem3/3(In3)
  Demux2/1 -> Subsystem/5(In5)

== system bit32cpu/ALU/Subsystem7/Subsystem4/Subsystem3 ==
  In1 : Inport
  In2 : Inport  Port=2
  In3 : Inport  Port=3
  In4 : Inport  Port=4
  In5 : Inport  Port=5
  In7 : Inport  Port=6
  In6 : Inport  Port=7
  Demux{,1..3} (4 alike) : Demux  Outputs=8
  Mux : Mux  Inputs=8
  Subsystem : Subsystem
  Subsystem1 : Subsystem
  Subsystem2 : Subsystem
  Subsystem3 : Subsystem
  Subsystem4 : Subsystem
  Subsystem5 : Subsystem
  Subsystem6 : Subsystem
  Subsystem7 : Subsystem
  Out1 : Outport
  wires:
  Demux3/7 -> Subsystem6/6(In6)
  In6/1 -> Subsystem4/7(In7), Subsystem7/7(In7), Subsystem5/7(In7), Subsystem6/7(In7), Subsystem1/7(In7), Subsystem3/7(In7), Subsystem2/7(In7), Subsystem/7(In7)
  Subsystem3/1(Out1) -> Mux/4
  Demux/1 -> Subsystem/3(In3)
  Demux2/8 -> Subsystem7/5(In5)
  Subsystem1/1(Out1) -> Mux/2
  Subsystem2/1(Out1) -> Mux/3
  Subsystem4/1(Out1) -> Mux/5
  Demux1/2 -> Subsystem1/4(In4)
  Demux/6 -> Subsystem5/3(In3)
  In4/1 -> Demux1/1
  Demux2/7 -> Subsystem6/5(In5)
  In3/1 -> Demux/1
  Demux1/4 -> Subsystem3/4(In4)
  In2/1 -> Subsystem4/2(In2), Subsystem5/2(In2), Subsystem6/2(In2), Subsystem7/2(In2), Subsystem2/2(In2), Subsystem3/2(In2), Subsystem/2(In2), Subsystem1/2(In2)
  Demux3/3 -> Subsystem2/6(In6)
  Subsystem/1(Out1) -> Mux/1
  Subsystem5/1(Out1) -> Mux/6
  In7/1 -> Demux3/1
  Mux/1 -> Out1/1
  Demux/3 -> Subsystem2/3(In3)
  Demux1/8 -> Subsystem7/4(In4)
  Demux3/6 -> Subsystem5/6(In6)
  Demux3/1 -> Subsystem/6(In6)
  Demux3/2 -> Subsystem1/6(In6)
  Subsystem6/1(Out1) -> Mux/7
  Demux1/3 -> Subsystem2/4(In4)
  Demux2/4 -> Subsystem3/5(In5)
  Demux1/5 -> Subsystem4/4(In4)
  In1/1 -> Subsystem6/1(In1), Subsystem7/1(In1), Subsystem4/1(In1), Subsystem5/1(In1), Subsystem2/1(In1), Subsystem3/1(In1), Subsystem/1(In1), Subsystem1/1(In1)
  Demux1/1 -> Subsystem/4(In4)
  Demux3/4 -> Subsystem3/6(In6)
  Demux2/2 -> Subsystem1/5(In5)
  Demux2/6 -> Subsystem5/5(In5)
  Demux/2 -> Subsystem1/3(In3)
  Demux/7 -> Subsystem6/3(In3)
  Demux3/8 -> Subsystem7/6(In6)
  Demux1/6 -> Subsystem5/4(In4)
  Demux/5 -> Subsystem4/3(In3)
  Demux2/5 -> Subsystem4/5(In5)
  Demux/8 -> Subsystem7/3(In3)
  Demux2/3 -> Subsystem2/5(In5)
  Demux3/5 -> Subsystem4/6(In6)
  In5/1 -> Demux2/1
  Demux1/7 -> Subsystem6/4(In4)
  Subsystem7/1(Out1) -> Mux/8
  Demux/4 -> Subsystem3/3(In3)
  Demux2/1 -> Subsystem/5(In5)

== system bit32cpu/ALU/Subsystem7/Subsystem4/Subsystem4 ==
  In1 : Inport
  In2 : Inport  Port=2
  In3 : Inport  Port=3
  In4 : Inport  Port=4
  In5 : Inport  Port=5
  In7 : Inport  Port=6
  In6 : Inport  Port=7
  Demux{,1..3} (4 alike) : Demux  Outputs=8
  Mux : Mux  Inputs=8
  Subsystem : Subsystem
  Subsystem1 : Subsystem
  Subsystem2 : Subsystem
  Subsystem3 : Subsystem
  Subsystem4 : Subsystem
  Subsystem5 : Subsystem
  Subsystem6 : Subsystem
  Subsystem7 : Subsystem
  Out1 : Outport
  wires:
  Demux3/7 -> Subsystem6/6(In6)
  In6/1 -> Subsystem4/7(In7), Subsystem7/7(In7), Subsystem5/7(In7), Subsystem6/7(In7), Subsystem1/7(In7), Subsystem3/7(In7), Subsystem2/7(In7), Subsystem/7(In7)
  Subsystem3/1(Out1) -> Mux/4
  Demux/1 -> Subsystem/3(In3)
  Demux2/8 -> Subsystem7/5(In5)
  Subsystem1/1(Out1) -> Mux/2
  Subsystem2/1(Out1) -> Mux/3
  Subsystem4/1(Out1) -> Mux/5
  Demux1/2 -> Subsystem1/4(In4)
  Demux/6 -> Subsystem5/3(In3)
  In4/1 -> Demux1/1
  Demux2/7 -> Subsystem6/5(In5)
  In3/1 -> Demux/1
  Demux1/4 -> Subsystem3/4(In4)
  In2/1 -> Subsystem4/2(In2), Subsystem5/2(In2), Subsystem6/2(In2), Subsystem7/2(In2), Subsystem2/2(In2), Subsystem3/2(In2), Subsystem/2(In2), Subsystem1/2(In2)
  Demux3/3 -> Subsystem2/6(In6)
  Subsystem/1(Out1) -> Mux/1
  Subsystem5/1(Out1) -> Mux/6
  In7/1 -> Demux3/1
  Mux/1 -> Out1/1
  Demux/3 -> Subsystem2/3(In3)
  Demux1/8 -> Subsystem7/4(In4)
  Demux3/6 -> Subsystem5/6(In6)
  Demux3/1 -> Subsystem/6(In6)
  Demux3/2 -> Subsystem1/6(In6)
  Subsystem6/1(Out1) -> Mux/7
  Demux1/3 -> Subsystem2/4(In4)
  Demux2/4 -> Subsystem3/5(In5)
  Demux1/5 -> Subsystem4/4(In4)
  In1/1 -> Subsystem6/1(In1), Subsystem7/1(In1), Subsystem4/1(In1), Subsystem5/1(In1), Subsystem2/1(In1), Subsystem3/1(In1), Subsystem/1(In1), Subsystem1/1(In1)
  Demux1/1 -> Subsystem/4(In4)
  Demux3/4 -> Subsystem3/6(In6)
  Demux2/2 -> Subsystem1/5(In5)
  Demux2/6 -> Subsystem5/5(In5)
  Demux/2 -> Subsystem1/3(In3)
  Demux/7 -> Subsystem6/3(In3)
  Demux3/8 -> Subsystem7/6(In6)
  Demux1/6 -> Subsystem5/4(In4)
  Demux/5 -> Subsystem4/3(In3)
  Demux2/5 -> Subsystem4/5(In5)
  Demux/8 -> Subsystem7/3(In3)
  Demux2/3 -> Subsystem2/5(In5)
  Demux3/5 -> Subsystem4/6(In6)
  In5/1 -> Demux2/1
  Demux1/7 -> Subsystem6/4(In4)
  Subsystem7/1(Out1) -> Mux/8
  Demux/4 -> Subsystem3/3(In3)
  Demux2/1 -> Subsystem/5(In5)

== system bit32cpu/ALU/Subsystem7/Subsystem4/Subsystem5 ==
  In1 : Inport
  In2 : Inport  Port=2
  In3 : Inport  Port=3
  In4 : Inport  Port=4
  In5 : Inport  Port=5
  In7 : Inport  Port=6
  In6 : Inport  Port=7
  Demux{,1..3} (4 alike) : Demux  Outputs=8
  Mux : Mux  Inputs=8
  Subsystem : Subsystem
  Subsystem1 : Subsystem
  Subsystem2 : Subsystem
  Subsystem3 : Subsystem
  Subsystem4 : Subsystem
  Subsystem5 : Subsystem
  Subsystem6 : Subsystem
  Subsystem7 : Subsystem
  Out1 : Outport
  wires:
  Demux3/7 -> Subsystem6/6(In6)
  In6/1 -> Subsystem4/7(In7), Subsystem7/7(In7), Subsystem5/7(In7), Subsystem6/7(In7), Subsystem1/7(In7), Subsystem3/7(In7), Subsystem2/7(In7), Subsystem/7(In7)
  Subsystem3/1(Out1) -> Mux/4
  Demux/1 -> Subsystem/3(In3)
  Demux2/8 -> Subsystem7/5(In5)
  Subsystem1/1(Out1) -> Mux/2
  Subsystem2/1(Out1) -> Mux/3
  Subsystem4/1(Out1) -> Mux/5
  Demux1/2 -> Subsystem1/4(In4)
  Demux/6 -> Subsystem5/3(In3)
  In4/1 -> Demux1/1
  Demux2/7 -> Subsystem6/5(In5)
  In3/1 -> Demux/1
  Demux1/4 -> Subsystem3/4(In4)
  In2/1 -> Subsystem4/2(In2), Subsystem5/2(In2), Subsystem6/2(In2), Subsystem7/2(In2), Subsystem2/2(In2), Subsystem3/2(In2), Subsystem/2(In2), Subsystem1/2(In2)
  Demux3/3 -> Subsystem2/6(In6)
  Subsystem/1(Out1) -> Mux/1
  Subsystem5/1(Out1) -> Mux/6
  In7/1 -> Demux3/1
  Mux/1 -> Out1/1
  Demux/3 -> Subsystem2/3(In3)
  Demux1/8 -> Subsystem7/4(In4)
  Demux3/6 -> Subsystem5/6(In6)
  Demux3/1 -> Subsystem/6(In6)
  Demux3/2 -> Subsystem1/6(In6)
  Subsystem6/1(Out1) -> Mux/7
  Demux1/3 -> Subsystem2/4(In4)
  Demux2/4 -> Subsystem3/5(In5)
  Demux1/5 -> Subsystem4/4(In4)
  In1/1 -> Subsystem6/1(In1), Subsystem7/1(In1), Subsystem4/1(In1), Subsystem5/1(In1), Subsystem2/1(In1), Subsystem3/1(In1), Subsystem/1(In1), Subsystem1/1(In1)
  Demux1/1 -> Subsystem/4(In4)
  Demux3/4 -> Subsystem3/6(In6)
  Demux2/2 -> Subsystem1/5(In5)
  Demux2/6 -> Subsystem5/5(In5)
  Demux/2 -> Subsystem1/3(In3)
  Demux/7 -> Subsystem6/3(In3)
  Demux3/8 -> Subsystem7/6(In6)
  Demux1/6 -> Subsystem5/4(In4)
  Demux/5 -> Subsystem4/3(In3)
  Demux2/5 -> Subsystem4/5(In5)
  Demux/8 -> Subsystem7/3(In3)
  Demux2/3 -> Subsystem2/5(In5)
  Demux3/5 -> Subsystem4/6(In6)
  In5/1 -> Demux2/1
  Demux1/7 -> Subsystem6/4(In4)
  Subsystem7/1(Out1) -> Mux/8
  Demux/4 -> Subsystem3/3(In3)
  Demux2/1 -> Subsystem/5(In5)

== system bit32cpu/ALU/Subtractor/Subtractor/Subsystem1 ==
  In1 : Inport
  In2 : Inport  Port=2
  In3 : Inport  Port=3
  Demux : Demux  Outputs=2
  Demux1 : Demux  Outputs=2
  Mux : Mux  Inputs=2
  Subsystem : Subsystem
  Subsystem1 : Subsystem
  Out1 : Outport
  Out2 : Outport  Port=2
  wires:
  Mux/1 -> Out2/1
  Subsystem1/2(Out2) -> Mux/1
  In2/1 -> Subsystem/2(In2)
  Subsystem1/1(Out1) -> Out1/1
  Demux/2 -> Subsystem/1(In1)
  In3/1 -> Demux1/1
  Demux1/2 -> Subsystem/3(In3)
  Demux/1 -> Subsystem1/1(In1)
  Demux1/1 -> Subsystem1/3(In3)
  In1/1 -> Demux/1
  Subsystem/2(Out2) -> Mux/2
  Subsystem/1(Out1) -> Subsystem1/2(In2)

== system bit32cpu/ALU/Subtractor/Subtractor/Subsystem2 ==
  In1 : Inport
  In2 : Inport  Port=2
  In3 : Inport  Port=3
  Demux : Demux  Outputs=2
  Demux1 : Demux  Outputs=2
  Mux : Mux  Inputs=2
  Subsystem : Subsystem
  Subsystem1 : Subsystem
  Out1 : Outport
  Out2 : Outport  Port=2
  wires:
  Mux/1 -> Out2/1
  Subsystem1/2(Out2) -> Mux/1
  In2/1 -> Subsystem/2(In2)
  Subsystem1/1(Out1) -> Out1/1
  Demux/2 -> Subsystem/1(In1)
  In3/1 -> Demux1/1
  Demux1/2 -> Subsystem/3(In3)
  Demux/1 -> Subsystem1/1(In1)
  Demux1/1 -> Subsystem1/3(In3)
  In1/1 -> Demux/1
  Subsystem/2(Out2) -> Mux/2
  Subsystem/1(Out1) -> Subsystem1/2(In2)

== system bit32cpu/ALU/Adder/Subsystem/Subsystem1/Subsystem ==
  In1 : Inport
  In2 : Inport  Port=2
  In3 : Inport  Port=3
  Demux : Demux  Outputs=2
  Demux1 : Demux  Outputs=2
  Mux : Mux  Inputs=2
  Subsystem1 : Subsystem
  Subsystem2 : Subsystem
  Out1 : Outport
  Out2 : Outport  Port=2
  wires:
  Subsystem2/1(Out1) -> Out1/1
  In3/1 -> Demux1/1
  Demux/1 -> Subsystem2/1(In1)
  Subsystem1/1(Out1) -> Subsystem2/2(In2)
  In2/1 -> Subsystem1/2(In2)
  In1/1 -> Demux/1
  Demux1/1 -> Subsystem2/3(In3)
  Mux/1 -> Out2/1
  Demux1/2 -> Subsystem1/3(In3)
  Demux/2 -> Subsystem1/1(In1)
  Subsystem2/2(Out2) -> Mux/1
  Subsystem1/2(Out2) -> Mux/2

== system bit32cpu/ALU/Adder/Subsystem/Subsystem1/Subsystem1 ==
  In1 : Inport
  In2 : Inport  Port=2
  In3 : Inport  Port=3
  Demux : Demux  Outputs=2
  Demux1 : Demux  Outputs=2
  Mux : Mux  Inputs=2
  Subsystem1 : Subsystem
  Subsystem2 : Subsystem
  Out1 : Outport
  Out2 : Outport  Port=2
  wires:
  Subsystem2/1(Out1) -> Out1/1
  In3/1 -> Demux1/1
  Demux/1 -> Subsystem2/1(In1)
  Subsystem1/1(Out1) -> Subsystem2/2(In2)
  In2/1 -> Subsystem1/2(In2)
  In1/1 -> Demux/1
  Demux1/1 -> Subsystem2/3(In3)
  Mux/1 -> Out2/1
  Demux1/2 -> Subsystem1/3(In3)
  Demux/2 -> Subsystem1/1(In1)
  Subsystem2/2(Out2) -> Mux/1
  Subsystem1/2(Out2) -> Mux/2

== system bit32cpu/ALU/Adder/Subsystem/Subsystem2/Subsystem ==
  In1 : Inport
  In2 : Inport  Port=2
  In3 : Inport  Port=3
  Demux : Demux  Outputs=2
  Demux1 : Demux  Outputs=2
  Mux : Mux  Inputs=2
  Subsystem1 : Subsystem
  Subsystem2 : Subsystem
  Out1 : Outport
  Out2 : Outport  Port=2
  wires:
  Subsystem2/1(Out1) -> Out1/1
  In3/1 -> Demux1/1
  Demux/1 -> Subsystem2/1(In1)
  Subsystem1/1(Out1) -> Subsystem2/2(In2)
  In2/1 -> Subsystem1/2(In2)
  In1/1 -> Demux/1
  Demux1/1 -> Subsystem2/3(In3)
  Mux/1 -> Out2/1
  Demux1/2 -> Subsystem1/3(In3)
  Demux/2 -> Subsystem1/1(In1)
  Subsystem2/2(Out2) -> Mux/1
  Subsystem1/2(Out2) -> Mux/2

== system bit32cpu/ALU/Adder/Subsystem/Subsystem2/Subsystem1 ==
  In1 : Inport
  In2 : Inport  Port=2
  In3 : Inport  Port=3
  Demux : Demux  Outputs=2
  Demux1 : Demux  Outputs=2
  Mux : Mux  Inputs=2
  Subsystem1 : Subsystem
  Subsystem2 : Subsystem
  Out1 : Outport
  Out2 : Outport  Port=2
  wires:
  Subsystem2/1(Out1) -> Out1/1
  In3/1 -> Demux1/1
  Demux/1 -> Subsystem2/1(In1)
  Subsystem1/1(Out1) -> Subsystem2/2(In2)
  In2/1 -> Subsystem1/2(In2)
  In1/1 -> Demux/1
  Demux1/1 -> Subsystem2/3(In3)
  Mux/1 -> Out2/1
  Demux1/2 -> Subsystem1/3(In3)
  Demux/2 -> Subsystem1/1(In1)
  Subsystem2/2(Out2) -> Mux/1
  Subsystem1/2(Out2) -> Mux/2

== system bit32cpu/ALU/Decrementer/Subtractor1/Subtractor/Subsystem1 ==
  In1 : Inport
  In2 : Inport  Port=2
  In3 : Inport  Port=3
  Demux : Demux  Outputs=2
  Demux1 : Demux  Outputs=2
  Mux : Mux  Inputs=2
  Subsystem : Subsystem
  Subsystem1 : Subsystem
  Out1 : Outport
  Out2 : Outport  Port=2
  wires:
  Mux/1 -> Out2/1
  Subsystem1/2(Out2) -> Mux/1
  In2/1 -> Subsystem/2(In2)
  Subsystem1/1(Out1) -> Out1/1
  Demux/2 -> Subsystem/1(In1)
  In3/1 -> Demux1/1
  Demux1/2 -> Subsystem/3(In3)
  Demux/1 -> Subsystem1/1(In1)
  Demux1/1 -> Subsystem1/3(In3)
  In1/1 -> Demux/1
  Subsystem/2(Out2) -> Mux/2
  Subsystem/1(Out1) -> Subsystem1/2(In2)

== system bit32cpu/ALU/Decrementer/Subtractor1/Subtractor/Subsystem2 ==
  In1 : Inport
  In2 : Inport  Port=2
  In3 : Inport  Port=3
  Demux : Demux  Outputs=2
  Demux1 : Demux  Outputs=2
  Mux : Mux  Inputs=2
  Subsystem : Subsystem
  Subsystem1 : Subsystem
  Out1 : Outport
  Out2 : Outport  Port=2
  wires:
  Mux/1 -> Out2/1
  Subsystem1/2(Out2) -> Mux/1
  In2/1 -> Subsystem/2(In2)
  Subsystem1/1(Out1) -> Out1/1
  Demux/2 -> Subsystem/1(In1)
  In3/1 -> Demux1/1
  Demux1/2 -> Subsystem/3(In3)
  Demux/1 -> Subsystem1/1(In1)
  Demux1/1 -> Subsystem1/3(In3)
  In1/1 -> Demux/1
  Subsystem/2(Out2) -> Mux/2
  Subsystem/1(Out1) -> Subsystem1/2(In2)

== system bit32cpu/ALU/Incrementer/Incrementer/Subsystem/Subsystem1 ==
  In1 : Inport
  In2 : Inport  Port=2
  In3 : Inport  Port=3
  Demux : Demux  Outputs=2
  Demux1 : Demux  Outputs=2
  Mux : Mux  Inputs=2
  Subsystem : Subsystem
  Subsystem1 : Subsystem
  Out1 : Outport
  Out2 : Outport  Port=2
  wires:
  Mux/1 -> Out2/1
  Subsystem1/2(Out2) -> Mux/1
  In2/1 -> Subsystem/2(In2)
  Subsystem1/1(Out1) -> Out1/1
  Demux/2 -> Subsystem/1(In1)
  In3/1 -> Demux1/1
  Demux1/2 -> Subsystem/3(In3)
  Demux/1 -> Subsystem1/1(In1)
  Demux1/1 -> Subsystem1/3(In3)
  In1/1 -> Demux/1
  Subsystem/2(Out2) -> Mux/2
  Subsystem/1(Out1) -> Subsystem1/2(In2)

== system bit32cpu/ALU/Incrementer/Incrementer/Subsystem/Subsystem2 ==
  In1 : Inport
  In2 : Inport  Port=2
  In3 : Inport  Port=3
  Demux : Demux  Outputs=2
  Demux1 : Demux  Outputs=2
  Mux : Mux  Inputs=2
  Subsystem : Subsystem
  Subsystem1 : Subsystem
  Out1 : Outport
  Out2 : Outport  Port=2
  wires:
  Mux/1 -> Out2/1
  Subsystem1/2(Out2) -> Mux/1
  In2/1 -> Subsystem/2(In2)
  Subsystem1/1(Out1) -> Out1/1
  Demux/2 -> Subsystem/1(In1)
  In3/1 -> Demux1/1
  Demux1/2 -> Subsystem/3(In3)
  Demux/1 -> Subsystem1/1(In1)
  Demux1/1 -> Subsystem1/3(In3)
  In1/1 -> Demux/1
  Subsystem/2(Out2) -> Mux/2
  Subsystem/1(Out1) -> Subsystem1/2(In2)

== system bit32cpu/ALU/Multiplier/Subsystem/Subsystem1/Subsystem ==
  In1 : Inport
  In2 : Inport  Port=2
  In3 : Inport  Port=3
  Demux : Demux  Outputs=2
  Demux1 : Demux  Outputs=2
  Mux : Mux  Inputs=2
  Subsystem1 : Subsystem
  Subsystem2 : Subsystem
  Out1 : Outport
  Out2 : Outport  Port=2
  wires:
  Subsystem2/1(Out1) -> Out1/1
  In3/1 -> Demux1/1
  Demux/1 -> Subsystem2/1(In1)
  Subsystem1/1(Out1) -> Subsystem2/2(In2)
  In2/1 -> Subsystem1/2(In2)
  In1/1 -> Demux/1
  Demux1/1 -> Subsystem2/3(In3)
  Mux/1 -> Out2/1
  Demux1/2 -> Subsystem1/3(In3)
  Demux/2 -> Subsystem1/1(In1)
  Subsystem2/2(Out2) -> Mux/1
  Subsystem1/2(Out2) -> Mux/2

== system bit32cpu/ALU/Multiplier/Subsystem/Subsystem1/Subsystem1 ==
  In1 : Inport
  In2 : Inport  Port=2
  In3 : Inport  Port=3
  Demux : Demux  Outputs=2
  Demux1 : Demux  Outputs=2
  Mux : Mux  Inputs=2
  Subsystem1 : Subsystem
  Subsystem2 : Subsystem
  Out1 : Outport
  Out2 : Outport  Port=2
  wires:
  Subsystem2/1(Out1) -> Out1/1
  In3/1 -> Demux1/1
  Demux/1 -> Subsystem2/1(In1)
  Subsystem1/1(Out1) -> Subsystem2/2(In2)
  In2/1 -> Subsystem1/2(In2)
  In1/1 -> Demux/1
  Demux1/1 -> Subsystem2/3(In3)
  Mux/1 -> Out2/1
  Demux1/2 -> Subsystem1/3(In3)
  Demux/2 -> Subsystem1/1(In1)
  Subsystem2/2(Out2) -> Mux/1
  Subsystem1/2(Out2) -> Mux/2

== system bit32cpu/ALU/Multiplier/Subsystem/Subsystem2/Subsystem ==
  In1 : Inport
  In2 : Inport  Port=2
  In3 : Inport  Port=3
  Demux : Demux  Outputs=2
  Demux1 : Demux  Outputs=2
  Mux : Mux  Inputs=2
  Subsystem1 : Subsystem
  Subsystem2 : Subsystem
  Out1 : Outport
  Out2 : Outport  Port=2
  wires:
  Subsystem2/1(Out1) -> Out1/1
  In3/1 -> Demux1/1
  Demux/1 -> Subsystem2/1(In1)
  Subsystem1/1(Out1) -> Subsystem2/2(In2)
  In2/1 -> Subsystem1/2(In2)
  In1/1 -> Demux/1
  Demux1/1 -> Subsystem2/3(In3)
  Mux/1 -> Out2/1
  Demux1/2 -> Subsystem1/3(In3)
  Demux/2 -> Subsystem1/1(In1)
  Subsystem2/2(Out2) -> Mux/1
  Subsystem1/2(Out2) -> Mux/2

== system bit32cpu/ALU/Multiplier/Subsystem/Subsystem2/Subsystem1 ==
  In1 : Inport
  In2 : Inport  Port=2
  In3 : Inport  Port=3
  Demux : Demux  Outputs=2
  Demux1 : Demux  Outputs=2
  Mux : Mux  Inputs=2
  Subsystem1 : Subsystem
  Subsystem2 : Subsystem
  Out1 : Outport
  Out2 : Outport  Port=2
  wires:
  Subsystem2/1(Out1) -> Out1/1
  In3/1 -> Demux1/1
  Demux/1 -> Subsystem2/1(In1)
  Subsystem1/1(Out1) -> Subsystem2/2(In2)
  In2/1 -> Subsystem1/2(In2)
  In1/1 -> Demux/1
  Demux1/1 -> Subsystem2/3(In3)
  Mux/1 -> Out2/1
  Demux1/2 -> Subsystem1/3(In3)
  Demux/2 -> Subsystem1/1(In1)
  Subsystem2/2(Out2) -> Mux/1
  Subsystem1/2(Out2) -> Mux/2

== system bit32cpu/ALU/Multiplier/Subsystem1/Subsystem/Subsystem5 ==
  In1 : Inport
  In2 : Inport  Port=2
  In3 : Inport  Port=3
  In4 : Inport  Port=4
  In5 : Inport  Port=5
  In6 : Inport  Port=6
  In7 : Inport  Port=7
  In8 : Inport  Port=8
  In17 : Inport  Port=9
  In9 : Inport  Port=10
  In10 : Inport  Port=11
  In11 : Inport  Port=12
  In12 : Inport  Port=13
  In13 : Inport  Port=14
  In14 : Inport  Port=15
  In15 : Inport  Port=16
  In16 : Inport  Port=17
  Subsystem : Subsystem
  Subsystem4 : Subsystem
  Out1 : Outport
  Out2 : Outport  Port=2
  Out3 : Outport  Port=3
  Out4 : Outport  Port=4
  Out5 : Outport  Port=5
  Out6 : Outport  Port=6
  Out7 : Outport  Port=7
  Out8 : Outport  Port=8
  Out9 : Outport  Port=9
  wires:
  Subsystem/3(Out3) -> Out7/1
  Subsystem4/5(Out5) -> Out5/1
  Subsystem4/3(Out3) -> Out3/1
  Subsystem4/1(Out1) -> Out1/1
  Subsystem/2(Out2) -> Out6/1
  Subsystem4/2(Out2) -> Out2/1
  Subsystem/1(Out1) -> Subsystem4/5(In5)
  Subsystem4/4(Out4) -> Out4/1
  Subsystem/5(Out5) -> Out9/1
  In17/1 -> Subsystem/5(In5)
  Subsystem/4(Out4) -> Out8/1
  In1/1 -> Subsystem4/1(In1)
  In2/1 -> Subsystem4/2(In2)
  In3/1 -> Subsystem4/3(In3)
  In4/1 -> Subsystem4/4(In4)
  In5/1 -> Subsystem/1(In1)
  In6/1 -> Subsystem/2(In2)
  In7/1 -> Subsystem/3(In3)
  In8/1 -> Subsystem/4(In4)
  In9/1 -> Subsystem4/6(In6)
  In10/1 -> Subsystem4/7(In7)
  In11/1 -> Subsystem4/8(In8)
  In12/1 -> Subsystem4/9(In9)
  In13/1 -> Subsystem/6(In6)
  In14/1 -> Subsystem/7(In7)
  In15/1 -> Subsystem/8(In8)
  In16/1 -> Subsystem/9(In9)

== system bit32cpu/ALU/Multiplier/Subsystem1/Subsystem/Subsystem6 ==
  In1 : Inport
  In2 : Inport  Port=2
  In3 : Inport  Port=3
  In4 : Inport  Port=4
  In5 : Inport  Port=5
  In6 : Inport  Port=6
  In7 : Inport  Port=7
  In8 : Inport  Port=8
  In9 : Inport  Port=9
  In10 : Inport  Port=10
  In11 : Inport  Port=11
  In12 : Inport  Port=12
  In13 : Inport  Port=13
  In14 : Inport  Port=14
  In15 : Inport  Port=15
  In16 : Inport  Port=16
  Constant16 : Constant  Value=0
  Subsystem : Subsystem
  Subsystem4 : Subsystem
  Out1 : Outport
  Out2 : Outport  Port=2
  Out3 : Outport  Port=3
  Out4 : Outport  Port=4
  Out5 : Outport  Port=5
  Out6 : Outport  Port=6
  Out7 : Outport  Port=7
  Out8 : Outport  Port=8
  Out9 : Outport  Port=9
  wires:
  Subsystem/3(Out3) -> Out7/1
  Subsystem4/5(Out5) -> Out5/1
  Subsystem4/3(Out3) -> Out3/1
  Subsystem4/1(Out1) -> Out1/1
  Subsystem/2(Out2) -> Out6/1
  Subsystem4/2(Out2) -> Out2/1
  Subsystem/1(Out1) -> Subsystem4/5(In5)
  Subsystem4/4(Out4) -> Out4/1
  Subsystem/5(Out5) -> Out9/1
  Constant16/1 -> Subsystem/5(In5)
  Subsystem/4(Out4) -> Out8/1
  In1/1 -> Subsystem4/1(In1)
  In2/1 -> Subsystem4/2(In2)
  In3/1 -> Subsystem4/3(In3)
  In4/1 -> Subsystem4/4(In4)
  In5/1 -> Subsystem/1(In1)
  In6/1 -> Subsystem/2(In2)
  In7/1 -> Subsystem/3(In3)
  In8/1 -> Subsystem/4(In4)
  In9/1 -> Subsystem4/6(In6)
  In10/1 -> Subsystem4/7(In7)
  In11/1 -> Subsystem4/8(In8)
  In12/1 -> Subsystem4/9(In9)
  In13/1 -> Subsystem/6(In6)
  In14/1 -> Subsystem/7(In7)
  In15/1 -> Subsystem/8(In8)
  In16/1 -> Subsystem/9(In9)
